simulink model "MOD4_A"  (Simulink 5.0)
settings: Solver=ode45  StartTime=0.0  StopTime=10.0  RelTol=1e-3
libraries: cstblocks x3, simulink_extras x1
settings Model: LastModifiedBy=ANNA  BlockReductionOpt=off  BooleanDataType=off

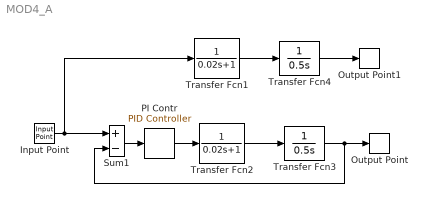
== system MOD4_A ==
  Input Point : cstblocks/Input Point
  Output Point : cstblocks/Output Point
  Output Point1 : cstblocks/Output Point
  PI Contr : simulink_extras/Additional Linear/PID Controller  P=12.5  I=150  D=0.
  Sum1 : Sum  Inputs=+-  SaturateOnIntegerOverflow=on  InputSameDT=on
  Transfer Fcn1 : TransferFcn  Denominator=[ 0.02 1]
  Transfer Fcn2 : TransferFcn  Denominator=[ 0.02 1]
  Transfer Fcn3 : TransferFcn  Denominator=[ 0.5 0]
  Transfer Fcn4 : TransferFcn  Denominator=[ 0.5 0]
  wires:
  Input Point/1 -> Sum1/1, Transfer Fcn1/1
  Sum1/1 -> PI Contr/1
  PI Contr/1 -> Transfer Fcn2/1
  Transfer Fcn2/1 -> Transfer Fcn3/1
  Transfer Fcn3/1 -> Sum1/2, Output Point/1
  Transfer Fcn1/1 -> Transfer Fcn4/1
  Transfer Fcn4/1 -> Output Point1/1
